simulink model "afti16sim"  (Simulink 5.0)
settings: Solver=ode45  SolverMode=SingleTasking  StartTime=0.0  StopTime=Tstop  RelTol=1e-3
values from neighbouring files (symbols this model uses):
  A = [-.0151 -60.5651 0 -32.174 ... (first row only)    [afti16.m]    (also in hessianNormalquadprog2D.m = [-0.5, 0, 0, 0; mpctry.m = [-0.5 1; 1 0]; quadprog15D.m = [-0.5 0; 1 0]; quadprog1D.m = [-0.5 0; 1 0])
  B = [-2.516 -13.136 ... (first row only)    [afti16.m]    (also in hessianNormalquadprog2D.m = [9.81, 0; mpctry.m = [9.81; 0]; quadprog15D.m = [9.81; 0]; quadprog1D.m = [9.81; 0])
  C = [0 1 0 0 ... (first row only)    [afti16.m]    (also in hessianNormalquadprog2D.m = [0, 1, 0, 1]; mpctry.m = [0, 1]; quadprog15D.m = [0, 1]; quadprog1D.m = [0, 1])
  Cf16e = expcon(Cf16,range,options)    [afti16.m]
  D = [0 0 ... (first row only)    [afti16.m]    (also in hessianNormalquadprog2D.m = [0, 0]; mpctry.m = [0]; quadprog15D.m = [0]; quadprog1D.m = [0])
  x0 = zeros(4,1)    [afti16.m]    (also in anoosh_pontyargin.m = [-0.5;0]; hessianNormalquadprog2D.m = [vel0(1); pos0(1); vel0(2); pos0(2)]; mpctry.m = [0, -0.5]; quadprog15D.m = [vel0(2); pos0(2)])
libraries: hyblib x1
settings Model: LastModifiedBy=Alberto Bemporad  ExtModeTrigMode=oneshot  ExtModeArmWhenConnect=off  LimitDataPoints=off  IntegerOverflowMsg=none  BooleanDataType=off

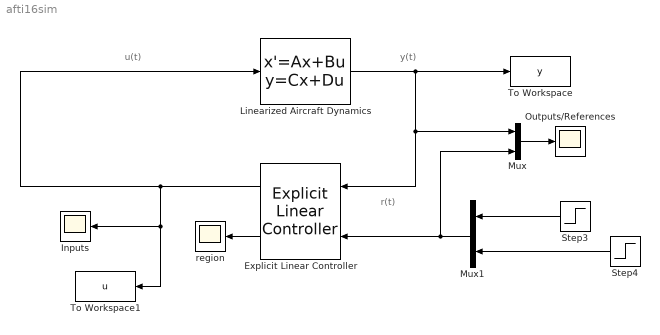
== system afti16sim ==
  note: u(t)
  note: y(t)
  note: r(t)
  Explicit Linear Controller : hyblib/Explicit Linear Controller  Orientation=left  C=Cf16e  xhat0=[]  u1=[]  compile=on
  Inputs : Scope
      settings: TimeRange=2  YMin=-30  YMax=30  DataFormat=Structure
  Linearized Aircraft Dynamics : StateSpace  A=A  B=B  C=C  D=D  X0=x0
  Mux : Mux  Inputs=2
  Mux1 : Mux  Orientation=left  Inputs=2
  Outputs/References : Scope
      settings: TimeRange=2  YMax=15  DataFormat=Structure
  Step3 : Step  Orientation=left  Time=0  After=0  SampleTime=0
  Step4 : Step  Orientation=left  Time=0  After=10  SampleTime=0
  To Workspace : ToWorkspace  VariableName=y  SampleTime=-1  SaveFormat=Array
  To Workspace1 : ToWorkspace  VariableName=u  SampleTime=-1  SaveFormat=Array
  region : Scope
      settings: TimeRange=2  YMin=0  YMax=15  DataFormat=Structure
  wires:
  Linearized Aircraft Dynamics/1 -> To Workspace/1, Mux/1, Explicit Linear Controller/1
  Mux/1 -> Outputs/References/1
  Explicit Linear Controller/1 -> Inputs/1, To Workspace1/1, Linearized Aircraft Dynamics/1
  Step3/1 -> Mux1/1
  Step4/1 -> Mux1/2
  Mux1/1 -> Mux/2, Explicit Linear Controller/2
  Explicit Linear Controller/2 -> region/1
